simulink model "ES003A_PwrDiscnct"  (R2013b)
settings: Solver=ode45  StartTime=0.0  StopTime=5  RelTol=1e-3
values from neighbouring files (symbols this model uses):
  BattVltgSwdMax = DataDict.Calibration    [ES250A_BattVltg_DataDict.m]
  ELECGLBPRM_IVTRCNT_CNT_U08 = DataDict.ConfigParam    [ES999A_ElecGlbPrm_DataDict.m]
  PwrDiscnctNtc0x042FailStep = DataDict.Calibration    [ES003A_PwrDiscnct_DataDict.m]
  PwrDiscnctNtc0x042PassStep = DataDict.Calibration    [ES003A_PwrDiscnct_DataDict.m]
  PwrDiscnctNtc0x04AFailStep = DataDict.Calibration    [ES003A_PwrDiscnct_DataDict.m]
  PwrDiscnctNtc0x04APassStep = DataDict.Calibration    [ES003A_PwrDiscnct_DataDict.m]
  PwrDiscnctOpenThd = DataDict.Calibration    [ES003A_PwrDiscnct_DataDict.m]
libraries: simulink x1
settings Model: Creator=BZ9NJH  LastModifiedBy=BZ9NJH

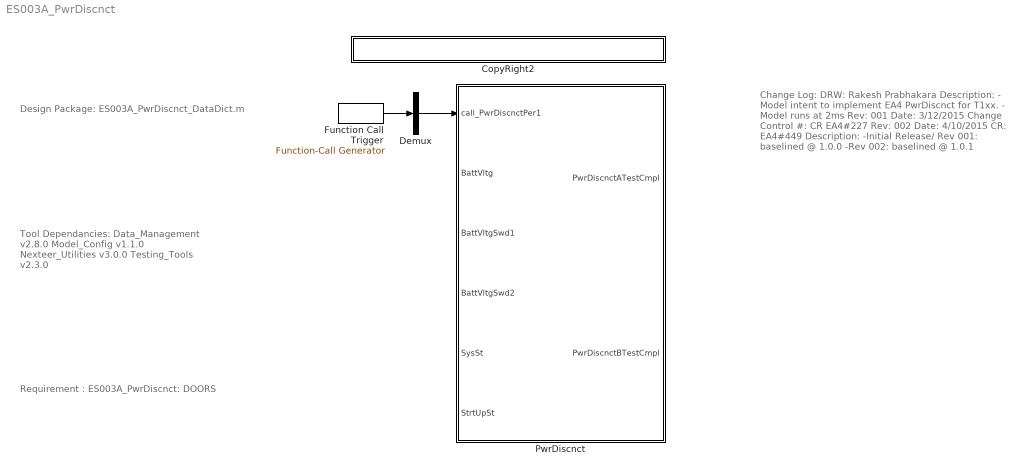
== system ES003A_PwrDiscnct ==
  note: Change Log:
      |
      | DRW: Rakesh Prabhakara
      | Description:
      | - Model intent to implement EA4 PwrDiscnct for T1xx.
      | - Model runs at 2ms
      |
      |
      | Rev: 001
      | Date: 3/12/2015
      | Change Control #: CR EA4#227
      |
      | Rev: 002
      | Date: 4/10/2015
      | CR: EA4#449
      |
      | Description:
      | -Initial Release/ Rev 001: baselined @ 1.0.0
      | -Rev 002: baselined @ 1.0.1
  note: Tool Dependancies:
      |
      | Data_Management v2.8.0
      | Model_Config v1.1.0
      | Nexteer_Utilities v3.0.0
      | Testing_Tools v2.3.0
  note: Design Package:
      |
      | ES003A_PwrDiscnct_DataDict.m
  note: Requirement :
      |
      | ES003A_PwrDiscnct: DOORS
  CopyRight2 : Subsystem  Description=|  mask(Copyright Information){none=on}
      | Copyright info block.                                               
      |                                                                     
      | Place copyright information at the top of every subsystem in design.
      mask prompts: none "No parameters"
      mask help: Place copyright information at the top of every subsystem in design.
      mask Display:
      | NxtrConf = 'Nexteer Confidential';
      | 
      | sys = bdroot; %handle for the current model ("system")
      | first = get_param(sys,'Created');
      | first = first(end-3:end);  %year is last four digits
      | 
      | last = get_param(sys,'LastModifiedDate');
      | if isempty(last)
      |     last = datestr(now,'yyyy');
      | else
      |     last = last(end-3:end);
      | end
      | 
      | if strcmp(first,last)
      |     fprintf('%s -- Copyright %s Nexteer',NxtrConf,first)
      | else
      |     fprintf('%s -- %s%s- %s Nexteer',NxtrConf,char(169),first,last)
      | end
  Demux : Demux  Outputs=1
  Function Call Trigger : simulink/Ports & Subsystems/Function-Call Generator  RequirementInfo={} %GIDa_15f970c6_0b7b_4174_a0b6_3f49a401e1d8  sample_time=0.002  numberOfIterations=1
  PwrDiscnct : Subsystem
  wires:
  Function Call Trigger/1 -> Demux/1
  Demux/1 -> PwrDiscnct/1(call_PwrDiscnctPer1)

== system ES003A_PwrDiscnct/CopyRight2 ==

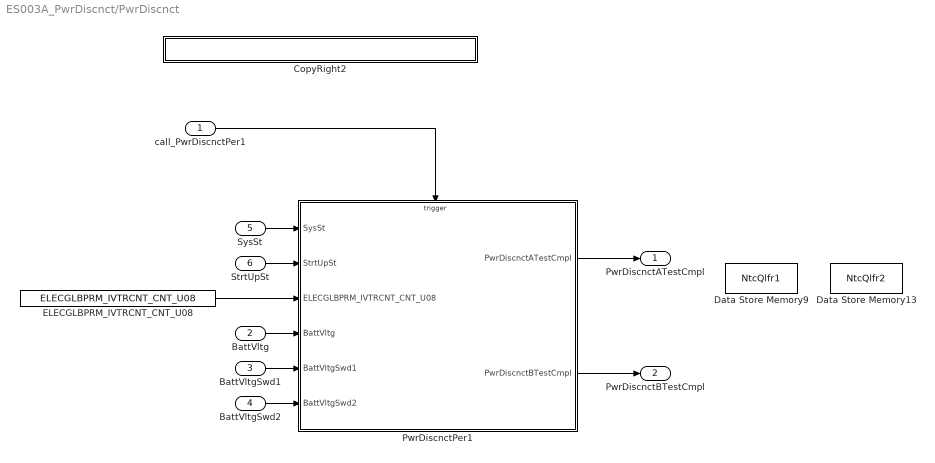
== system ES003A_PwrDiscnct/PwrDiscnct ==
  call_PwrDiscnctPer1 : Inport
  BattVltg : Inport  RequirementInfo={'linktype_rmi_doors' '0000c467 (/ESG Group/FDD Module Requirements/EA4 Specific/ES003A_PwrDiscnct)' '#ES003A_10' 'true' 'REQ: ES003A_10' '' } %GIDa_7969af00_7b99_4bd8_ab11_a14ecd32b67f  Port=2
  BattVltgSwd1 : Inport  RequirementInfo={'linktype_rmi_doors' '0000c467 (/ESG Group/FDD Module Requirements/EA4 Specific/ES003A_PwrDiscnct)' '#ES003A_11' 'true' 'REQ: ES003A_11' '' } %GIDa_b2ae44ec_3256_4720_9bec_d529845afe91  Port=3
  BattVltgSwd2 : Inport  RequirementInfo={'linktype_rmi_doors' '0000c467 (/ESG Group/FDD Module Requirements/EA4 Specific/ES003A_PwrDiscnct)' '#ES003A_12' 'true' 'REQ: ES003A_12' '' } %GIDa_6e68fbbb_22b3_47e1_b135_14c1a3669e24  Port=4
  SysSt : Inport  Port=5
  StrtUpSt : Inport  RequirementInfo={'linktype_rmi_doors' '0000c467 (/ESG Group/FDD Module Requirements/EA4 Specific/ES003A_PwrDiscnct)' '#ES003A_106' 'true' 'REQ: ES003A_106' '' } %GIDa_3a5ffb6b_2c5b_4987_b033_10885cd35b25  Port=6  OutDataTypeStr=double
  CopyRight2 : Subsystem  Description=|  mask(Copyright Information){none=on}
      | Copyright info block.                                               
      |                                                                     
      | Place copyright information at the top of every subsystem in design.
      mask prompts: none "No parameters"
      mask help: Place copyright information at the top of every subsystem in design.
      mask Display:
      | NxtrConf = 'Nexteer Confidential';
      | 
      | sys = bdroot; %handle for the current model ("system")
      | first = get_param(sys,'Created');
      | first = first(end-3:end);  %year is last four digits
      | 
      | last = get_param(sys,'LastModifiedDate');
      | if isempty(last)
      |     last = datestr(now,'yyyy');
      | else
      |     last = last(end-3:end);
      | end
      | 
      | if strcmp(first,last)
      |     fprintf('%s -- Copyright %s Nexteer',NxtrConf,first)
      | else
      |     fprintf('%s -- %s%s- %s Nexteer',NxtrConf,char(169),first,last)
      | end
  Data Store Memory13 : DataStoreMemory  DataStoreName=NtcQlfr2  ReadBeforeWriteMsg=warning  WriteAfterWriteMsg=warning  WriteAfterReadMsg=warning
  Data Store Memory9 : DataStoreMemory  DataStoreName=NtcQlfr1  ReadBeforeWriteMsg=warning  WriteAfterWriteMsg=warning  WriteAfterReadMsg=warning
  ELECGLBPRM_IVTRCNT_CNT_U08 : Constant  RequirementInfo={'linktype_rmi_doors' '0000c467 (/ESG Group/FDD Module Requirements/EA4 Specific/ES003A_PwrDiscnct)' '#ES003A_13' 'true' 'REQ: ES003A_13' '' } %GIDa_8c2aeced_6f98_4fdd_a2dd_374f750473e0  Value=ELECGLBPRM_IVTRCNT_CNT_U08  OutDataTypeStr=single
  PwrDiscnctPer1 : Subsystem  RequirementInfo={'linktype_rmi_doors' '0000c467 (/ESG Group/FDD Module Requirements/EA4 Specific/ES003A_PwrDiscnct)' '#ES003A_98' 'true' 'REQ: ES003A_98' '' } %GIDa_d6496f46_22fb_4d18_9ef4_8fee2b8599d6  TreatAsAtomicUnit=on
  PwrDiscnctATestCmpl : Outport  RequirementInfo={'linktype_rmi_doors' '0000c467 (/ESG Group/FDD Module Requirements/EA4 Specific/ES003A_PwrDiscnct)' '#ES003A_15' 'true' 'REQ: ES003A_15' '' } %GIDa_a54f22bb_d830_4888_91ed_92219a6abd25
  PwrDiscnctBTestCmpl : Outport  RequirementInfo={'linktype_rmi_doors' '0000c467 (/ESG Group/FDD Module Requirements/EA4 Specific/ES003A_PwrDiscnct)' '#ES003A_14' 'true' 'REQ: ES003A_14' '' } %GIDa_e99709b4_314c_405c_b628_2ebeb252bf18  Port=2
  wires:
  call_PwrDiscnctPer1/1 -> PwrDiscnctPer1/Trigger
  PwrDiscnctPer1/1(PwrDiscnctATestCmpl) -> PwrDiscnctATestCmpl/1
  PwrDiscnctPer1/2(PwrDiscnctBTestCmpl) -> PwrDiscnctBTestCmpl/1
  StrtUpSt/1 -> PwrDiscnctPer1/2(StrtUpSt)
  SysSt/1 -> PwrDiscnctPer1/1(SysSt)
  ELECGLBPRM_IVTRCNT_CNT_U08/1 -> PwrDiscnctPer1/3(ELECGLBPRM_IVTRCNT_CNT_U08)
  BattVltg/1 -> PwrDiscnctPer1/4(BattVltg)
  BattVltgSwd2/1 -> PwrDiscnctPer1/6(BattVltgSwd2)
  BattVltgSwd1/1 -> PwrDiscnctPer1/5(BattVltgSwd1)

== system ES003A_PwrDiscnct/PwrDiscnct/CopyRight2 ==

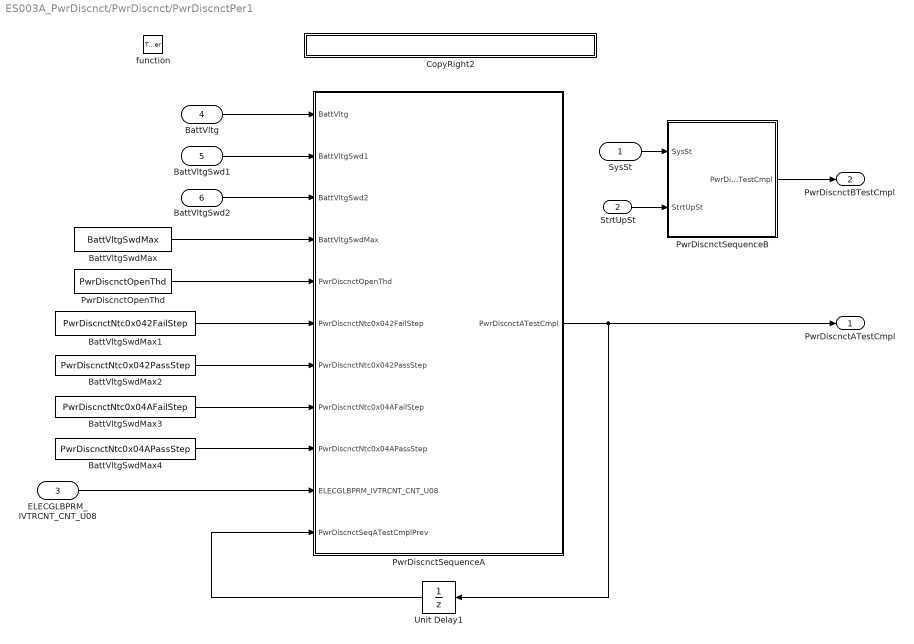
== system ES003A_PwrDiscnct/PwrDiscnct/PwrDiscnctPer1 ==
  SysSt : Inport
  StrtUpSt : Inport  Port=2  OutDataTypeStr=double
  ELECGLBPRM_IVTRCNT_CNT_U08 : Inport  Port=3
  BattVltg : Inport  Port=4
  BattVltgSwd1 : Inport  Port=5
  BattVltgSwd2 : Inport  Port=6
  function : TriggerPort  TriggerType=function-call
  BattVltgSwdMax : Constant  RequirementInfo={'linktype_rmi_doors' '0000c467 (/ESG Group/FDD Module Requirements/EA4 Specific/ES003A_PwrDiscnct)' '#ES003A_18' 'true' 'REQ: ES003A_18' '' } %GIDa_75c0cbae_266b_43df_b9ef_273f9bdf4671  Value=BattVltgSwdMax
  BattVltgSwdMax1 : Constant  Value=PwrDiscnctNtc0x042FailStep
  BattVltgSwdMax2 : Constant  Value=PwrDiscnctNtc0x042PassStep
  BattVltgSwdMax3 : Constant  Value=PwrDiscnctNtc0x04AFailStep
  BattVltgSwdMax4 : Constant  Value=PwrDiscnctNtc0x04APassStep
  CopyRight2 : Subsystem  Description=|  mask(Copyright Information){none=on}
      | Copyright info block.                                               
      |                                                                     
      | Place copyright information at the top of every subsystem in design.
      mask prompts: none "No parameters"
      mask help: Place copyright information at the top of every subsystem in design.
      mask Display:
      | NxtrConf = 'Nexteer Confidential';
      | 
      | sys = bdroot; %handle for the current model ("system")
      | first = get_param(sys,'Created');
      | first = first(end-3:end);  %year is last four digits
      | 
      | last = get_param(sys,'LastModifiedDate');
      | if isempty(last)
      |     last = datestr(now,'yyyy');
      | else
      |     last = last(end-3:end);
      | end
      | 
      | if strcmp(first,last)
      |     fprintf('%s -- Copyright %s Nexteer',NxtrConf,first)
      | else
      |     fprintf('%s -- %s%s- %s Nexteer',NxtrConf,char(169),first,last)
      | end
  PwrDiscnctOpenThd : Constant  RequirementInfo={'linktype_rmi_doors' '0000c467 (/ESG Group/FDD Module Requirements/EA4 Specific/ES003A_PwrDiscnct)' '#ES003A_22' 'true' 'REQ: ES003A_22' '' } %GIDa_a84f9b62_e1cf_4caf_a19c_8d6c01e9295c  Value=PwrDiscnctOpenThd
  PwrDiscnctSequenceA : Stateflow chart  RequirementInfo={'linktype_rmi_doors' '0000c467 (/ESG Group/FDD Module Requirements/EA4 Specific/ES003A_PwrDiscnct)' '#ES003A_47' 'true' 'REQ: ES003A_47' '' } %GIDa_3ade2cbb_cb37_4d62_9bbf_15e89d094b58  TreatAsAtomicUnit=on
  PwrDiscnctSequenceB : Subsystem  RequirementInfo={'linktype_rmi_doors' '0000c467 (/ESG Group/FDD Module Requirements/EA4 Specific/ES003A_PwrDiscnct)' '#ES003A_82' 'true' 'REQ: ES003A_82' '' ; 'linktype_rmi_doors' '0000c467 (/ESG Group/FDD Module Requirements/EA4 Specific/ES003A_PwrDiscnct)' '#ES003A_88' 'true' 'REQ: ES003A_88' '' } %GIDa_af92003a_7581_41aa_9d02_d4566cd9fce6
  Unit Delay1 : UnitDelay  SampleTime=-1  StateName=PwrDiscnctSeqATestCmplPrev  StateMustResolveToSignalObject=on
      settings: AttributesFormatString=|
      | State Name:
      | %<StateName>
  PwrDiscnctATestCmpl : Outport
  PwrDiscnctBTestCmpl : Outport  Port=2
  wires:
  SysSt/1 -> PwrDiscnctSequenceB/1(SysSt)
  BattVltg/1 -> PwrDiscnctSequenceA/1(BattVltg)
  BattVltgSwd1/1 -> PwrDiscnctSequenceA/2(BattVltgSwd1)
  BattVltgSwd2/1 -> PwrDiscnctSequenceA/3(BattVltgSwd2)
  ELECGLBPRM_IVTRCNT_CNT_U08/1 -> PwrDiscnctSequenceA/10(ELECGLBPRM_IVTRCNT_CNT_U08)
  PwrDiscnctOpenThd/1 -> PwrDiscnctSequenceA/5(PwrDiscnctOpenThd)
  BattVltgSwdMax/1 -> PwrDiscnctSequenceA/4(BattVltgSwdMax)
  BattVltgSwdMax1/1 -> PwrDiscnctSequenceA/6(PwrDiscnctNtc0x042FailStep)
  BattVltgSwdMax2/1 -> PwrDiscnctSequenceA/7(PwrDiscnctNtc0x042PassStep)
  BattVltgSwdMax3/1 -> PwrDiscnctSequenceA/8(PwrDiscnctNtc0x04AFailStep)
  BattVltgSwdMax4/1 -> PwrDiscnctSequenceA/9(PwrDiscnctNtc0x04APassStep)
  PwrDiscnctSequenceA/1(PwrDiscnctATestCmpl) -> Unit Delay1/1, PwrDiscnctATestCmpl/1
  Unit Delay1/1 -> PwrDiscnctSequenceA/11(PwrDiscnctSeqATestCmplPrev)
  PwrDiscnctSequenceB/1(PwrDiscnctBTestCmpl) -> PwrDiscnctBTestCmpl/1
  StrtUpSt/1 -> PwrDiscnctSequenceB/2(StrtUpSt)

== system ES003A_PwrDiscnct/PwrDiscnct/PwrDiscnctPer1/CopyRight2 ==

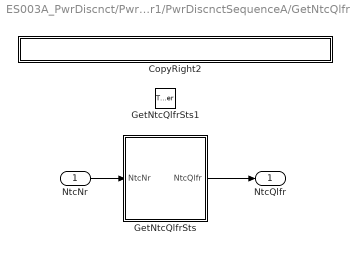
== system ES003A_PwrDiscnct/PwrDiscnct/PwrDiscnctPer1/PwrDiscnctSequenceA/GetNtcQlfrSts ==
  NtcNr : Inport  OutDataTypeStr=int16  PortDimensions=1
  GetNtcQlfrSts1 : TriggerPort  TriggerType=function-call
      settings: CopyFcn=Stateflow.SLINSF.SimulinkMan.removeBlockPreDeleteFcn  PreDeleteFcn=Stateflow.SLINSF.SimulinkMan.unsafePredeleteFcn
  CopyRight2 : Subsystem  Description=|  mask(Copyright Information){none=on}
      | Copyright info block.                                               
      |                                                                     
      | Place copyright information at the top of every subsystem in design.
      mask prompts: none "No parameters"
      mask help: Place copyright information at the top of every subsystem in design.
      mask Display:
      | NxtrConf = 'Nexteer Confidential';
      | 
      | sys = bdroot; %handle for the current model ("system")
      | first = get_param(sys,'Created');
      | first = first(end-3:end);  %year is last four digits
      | 
      | last = get_param(sys,'LastModifiedDate');
      | if isempty(last)
      |     last = datestr(now,'yyyy');
      | else
      |     last = last(end-3:end);
      | end
      | 
      | if strcmp(first,last)
      |     fprintf('%s -- Copyright %s Nexteer',NxtrConf,first)
      | else
      |     fprintf('%s -- %s%s- %s Nexteer',NxtrConf,char(169),first,last)
      | end
  GetNtcQlfrSts : Subsystem  RequirementInfo={} %GIDa_55b4ee3c_edbf_4f51_ae1c_660e8f62e0b1  TreatAsAtomicUnit=on
      settings: RTWSystemCode=Inline
  NtcQlfr : Outport
  wires:
  NtcNr/1 -> GetNtcQlfrSts/1(NtcNr)
  GetNtcQlfrSts/1(NtcQlfr) -> NtcQlfr/1

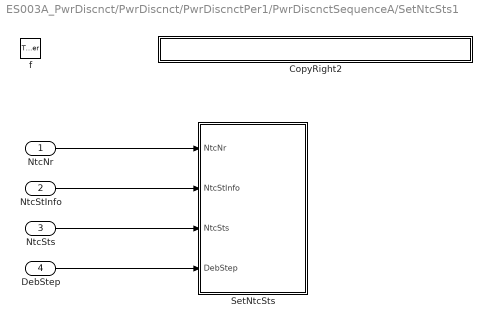
== system ES003A_PwrDiscnct/PwrDiscnct/PwrDiscnctPer1/PwrDiscnctSequenceA/SetNtcSts1 ==
  NtcNr : Inport  PortDimensions=1
  NtcStInfo : Inport  Port=2  PortDimensions=1
  NtcSts : Inport  Port=3  PortDimensions=1
  DebStep : Inport  Port=4  PortDimensions=1
  f : TriggerPort  TriggerType=function-call
      settings: CopyFcn=Stateflow.SLINSF.SimulinkMan.removeBlockPreDeleteFcn  PreDeleteFcn=Stateflow.SLINSF.SimulinkMan.unsafePredeleteFcn
  CopyRight2 : Subsystem  Description=|  mask(Copyright Information){none=on}
      | Copyright info block.                                               
      |                                                                     
      | Place copyright information at the top of every subsystem in design.
      mask prompts: none "No parameters"
      mask help: Place copyright information at the top of every subsystem in design.
      mask Display:
      | NxtrConf = 'Nexteer Confidential';
      | 
      | sys = bdroot; %handle for the current model ("system")
      | first = get_param(sys,'Created');
      | first = first(end-3:end);  %year is last four digits
      | 
      | last = get_param(sys,'LastModifiedDate');
      | if isempty(last)
      |     last = datestr(now,'yyyy');
      | else
      |     last = last(end-3:end);
      | end
      | 
      | if strcmp(first,last)
      |     fprintf('%s -- Copyright %s Nexteer',NxtrConf,first)
      | else
      |     fprintf('%s -- %s%s- %s Nexteer',NxtrConf,char(169),first,last)
      | end
  SetNtcSts : Subsystem  RequirementInfo={} %GIDa_82714b20_8369_498a_a3bf_ae484680a262  VariantControl=NTC_sim
  wires:
  NtcStInfo/1 -> SetNtcSts/2(NtcStInfo)
  NtcNr/1 -> SetNtcSts/1(NtcNr)
  NtcSts/1 -> SetNtcSts/3(NtcSts)
  DebStep/1 -> SetNtcSts/4(DebStep)

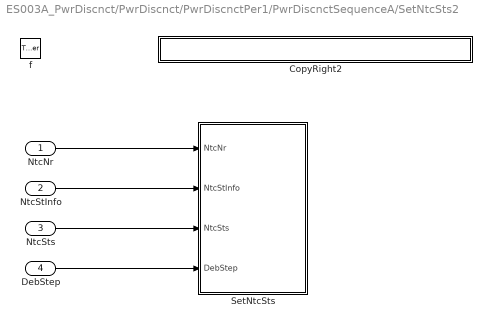
== system ES003A_PwrDiscnct/PwrDiscnct/PwrDiscnctPer1/PwrDiscnctSequenceA/SetNtcSts2 ==
  NtcNr : Inport  PortDimensions=1
  NtcStInfo : Inport  Port=2  PortDimensions=1
  NtcSts : Inport  Port=3  PortDimensions=1
  DebStep : Inport  Port=4  PortDimensions=1
  f : TriggerPort  TriggerType=function-call
      settings: CopyFcn=Stateflow.SLINSF.SimulinkMan.removeBlockPreDeleteFcn  PreDeleteFcn=Stateflow.SLINSF.SimulinkMan.unsafePredeleteFcn
  CopyRight2 : Subsystem  Description=|  mask(Copyright Information){none=on}
      | Copyright info block.                                               
      |                                                                     
      | Place copyright information at the top of every subsystem in design.
      mask prompts: none "No parameters"
      mask help: Place copyright information at the top of every subsystem in design.
      mask Display:
      | NxtrConf = 'Nexteer Confidential';
      | 
      | sys = bdroot; %handle for the current model ("system")
      | first = get_param(sys,'Created');
      | first = first(end-3:end);  %year is last four digits
      | 
      | last = get_param(sys,'LastModifiedDate');
      | if isempty(last)
      |     last = datestr(now,'yyyy');
      | else
      |     last = last(end-3:end);
      | end
      | 
      | if strcmp(first,last)
      |     fprintf('%s -- Copyright %s Nexteer',NxtrConf,first)
      | else
      |     fprintf('%s -- %s%s- %s Nexteer',NxtrConf,char(169),first,last)
      | end
  SetNtcSts : Subsystem  RequirementInfo={} %GIDa_0f1cc213_d07f_475f_8cac_6a7fd5400116  VariantControl=NTC_sim
  wires:
  NtcStInfo/1 -> SetNtcSts/2(NtcStInfo)
  NtcNr/1 -> SetNtcSts/1(NtcNr)
  NtcSts/1 -> SetNtcSts/3(NtcSts)
  DebStep/1 -> SetNtcSts/4(DebStep)

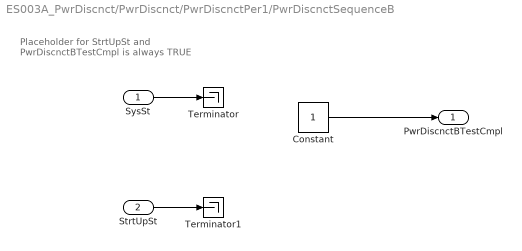
== system ES003A_PwrDiscnct/PwrDiscnct/PwrDiscnctPer1/PwrDiscnctSequenceB ==
  note: Placeholder for StrtUpSt
      | and  PwrDiscnctBTestCmpl is always TRUE
  SysSt : Inport
  StrtUpSt : Inport  Port=2
  Constant : Constant
  Terminator : Terminator
  Terminator1 : Terminator
  PwrDiscnctBTestCmpl : Outport
  wires:
  Constant/1 -> PwrDiscnctBTestCmpl/1
  SysSt/1 -> Terminator/1
  StrtUpSt/1 -> Terminator1/1

== system ES003A_PwrDiscnct/PwrDiscnct/PwrDiscnctPer1/PwrDiscnctSequenceA/GetNtcQlfrSts/CopyRight2 ==

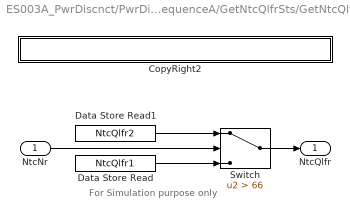
== system ES003A_PwrDiscnct/PwrDiscnct/PwrDiscnctPer1/PwrDiscnctSequenceA/GetNtcQlfrSts/GetNtcQlfrSts ==
  note: For Simulation purpose only
  NtcNr : Inport
  CopyRight2 : Subsystem  Description=|  mask(Copyright Information){none=on}
      | Copyright info block.                                               
      |                                                                     
      | Place copyright information at the top of every subsystem in design.
      mask prompts: none "No parameters"
      mask help: Place copyright information at the top of every subsystem in design.
      mask Display:
      | NxtrConf = 'Nexteer Confidential';
      | 
      | sys = bdroot; %handle for the current model ("system")
      | first = get_param(sys,'Created');
      | first = first(end-3:end);  %year is last four digits
      | 
      | last = get_param(sys,'LastModifiedDate');
      | if isempty(last)
      |     last = datestr(now,'yyyy');
      | else
      |     last = last(end-3:end);
      | end
      | 
      | if strcmp(first,last)
      |     fprintf('%s -- Copyright %s Nexteer',NxtrConf,first)
      | else
      |     fprintf('%s -- %s%s- %s Nexteer',NxtrConf,char(169),first,last)
      | end
  Data Store Read : DataStoreRead  DataStoreName=NtcQlfr1
  Data Store Read1 : DataStoreRead  DataStoreName=NtcQlfr2
  Switch : Switch  Criteria=u2 > Threshold  Threshold=66
  NtcQlfr : Outport
  wires:
  Switch/1 -> NtcQlfr/1
  NtcNr/1 -> Switch/2
  Data Store Read1/1 -> Switch/1
  Data Store Read/1 -> Switch/3

== system ES003A_PwrDiscnct/PwrDiscnct/PwrDiscnctPer1/PwrDiscnctSequenceA/SetNtcSts1/CopyRight2 ==

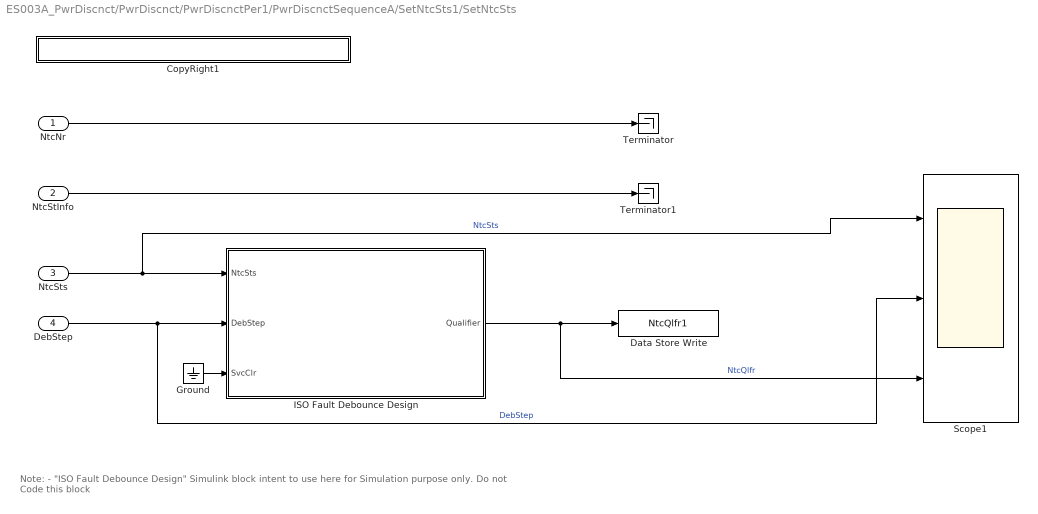
== system ES003A_PwrDiscnct/PwrDiscnct/PwrDiscnctPer1/PwrDiscnctSequenceA/SetNtcSts1/SetNtcSts ==
  note: Note:
      |
      | - "ISO Fault Debounce Design" Simulink block intent to use here for Simulation purpose only. Do not Code this block
  NtcNr : Inport
  NtcStInfo : Inport  Port=2
  NtcSts : Inport  Port=3
  DebStep : Inport  Port=4
  CopyRight1 : Subsystem  Description=|  mask(Copyright Information){none=on}
      | Copyright info block.                                               
      |                                                                     
      | Place copyright information at the top of every subsystem in design.
      mask prompts: none "No parameters"
      mask help: Place copyright information at the top of every subsystem in design.
      mask Display:
      | NxtrConf = 'Nexteer Confidential';
      | 
      | sys = bdroot; %handle for the current model ("system")
      | first = get_param(sys,'Created');
      | first = first(end-3:end);  %year is last four digits
      | 
      | last = get_param(sys,'LastModifiedDate');
      | if isempty(last)
      |     last = datestr(now,'yyyy');
      | else
      |     last = last(end-3:end);
      | end
      | 
      | if strcmp(first,last)
      |     fprintf('%s -- Copyright %s Nexteer',NxtrConf,first)
      | else
      |     fprintf('%s -- %s%s- %s Nexteer',NxtrConf,char(169),first,last)
      | end
  Data Store Write : DataStoreWrite  DataStoreName=NtcQlfr1
  Ground : Ground
  ISO Fault Debounce Design : Stateflow chart  TreatAsAtomicUnit=on
      settings: AttributesFormatString=|
      | Simulation Purpose Only.
      | Do Not Code this block
      | Diagnostic Manager Owns this requirement
  Scope1 : Scope  NumInputPorts=3
      settings: YMin=1.9~3891.2~-1  YMax=2.1~4300.8~1
  Terminator : Terminator
  Terminator1 : Terminator
  wires:
  NtcStInfo/1 -> Terminator1/1
  NtcNr/1 -> Terminator/1
  NtcSts/1 -> ISO Fault Debounce Design/1(NtcSts), Scope1/1  "NtcSts"
  DebStep/1 -> ISO Fault Debounce Design/2(DebStep), Scope1/2  "DebStep"
  ISO Fault Debounce Design/1(Qualifier) -> Scope1/3, Data Store Write/1  "NtcQlfr"
  Ground/1 -> ISO Fault Debounce Design/3(SvcClr)

== system ES003A_PwrDiscnct/PwrDiscnct/PwrDiscnctPer1/PwrDiscnctSequenceA/SetNtcSts2/CopyRight2 ==

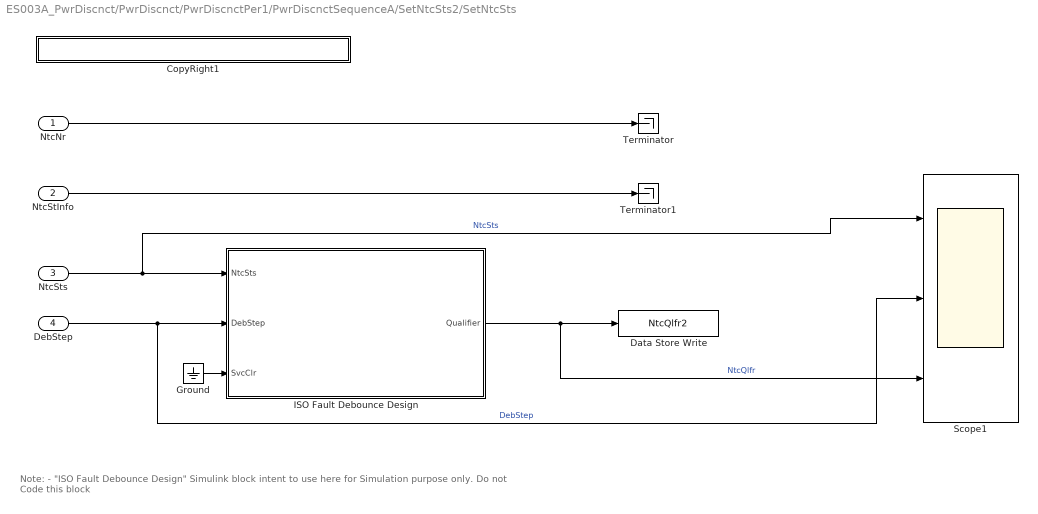
== system ES003A_PwrDiscnct/PwrDiscnct/PwrDiscnctPer1/PwrDiscnctSequenceA/SetNtcSts2/SetNtcSts ==
  note: Note:
      |
      | - "ISO Fault Debounce Design" Simulink block intent to use here for Simulation purpose only. Do not Code this block
  NtcNr : Inport
  NtcStInfo : Inport  Port=2
  NtcSts : Inport  Port=3
  DebStep : Inport  Port=4
  CopyRight1 : Subsystem  Description=|  mask(Copyright Information){none=on}
      | Copyright info block.                                               
      |                                                                     
      | Place copyright information at the top of every subsystem in design.
      mask prompts: none "No parameters"
      mask help: Place copyright information at the top of every subsystem in design.
      mask Display:
      | NxtrConf = 'Nexteer Confidential';
      | 
      | sys = bdroot; %handle for the current model ("system")
      | first = get_param(sys,'Created');
      | first = first(end-3:end);  %year is last four digits
      | 
      | last = get_param(sys,'LastModifiedDate');
      | if isempty(last)
      |     last = datestr(now,'yyyy');
      | else
      |     last = last(end-3:end);
      | end
      | 
      | if strcmp(first,last)
      |     fprintf('%s -- Copyright %s Nexteer',NxtrConf,first)
      | else
      |     fprintf('%s -- %s%s- %s Nexteer',NxtrConf,char(169),first,last)
      | end
  Data Store Write : DataStoreWrite  DataStoreName=NtcQlfr2
  Ground : Ground
  ISO Fault Debounce Design : Stateflow chart  TreatAsAtomicUnit=on
      settings: AttributesFormatString=|
      | Simulation Purpose Only.
      | Do Not Code this block
      | Diagnostic Manager Owns this requirement
  Scope1 : Scope  NumInputPorts=3
      settings: YMin=1.9~486.4~0  YMax=2.1~537.6~1
  Terminator : Terminator
  Terminator1 : Terminator
  wires:
  NtcStInfo/1 -> Terminator1/1
  NtcNr/1 -> Terminator/1
  NtcSts/1 -> ISO Fault Debounce Design/1(NtcSts), Scope1/1  "NtcSts"
  DebStep/1 -> ISO Fault Debounce Design/2(DebStep), Scope1/2  "DebStep"
  ISO Fault Debounce Design/1(Qualifier) -> Scope1/3, Data Store Write/1  "NtcQlfr"
  Ground/1 -> ISO Fault Debounce Design/3(SvcClr)

== system ES003A_PwrDiscnct/PwrDiscnct/PwrDiscnctPer1/PwrDiscnctSequenceA/GetNtcQlfrSts/GetNtcQlfrSts/CopyRight2 ==

== system ES003A_PwrDiscnct/PwrDiscnct/PwrDiscnctPer1/PwrDiscnctSequenceA/SetNtcSts1/SetNtcSts/CopyRight1 ==

== system ES003A_PwrDiscnct/PwrDiscnct/PwrDiscnctPer1/PwrDiscnctSequenceA/SetNtcSts2/SetNtcSts/CopyRight1 ==

== stateflow chart ES003A_PwrDiscnct/PwrDiscnct/PwrDiscnctPer1/PwrDiscnctSequenceA ==
  state SetNtcSts1(NtcNr, NtcStInfo, NtcSts, DebStep) [function]
  state NtcQlfr = GetNtcQlfrSts(NtcNr) [function]
  state SetNtcSts2(NtcNr, NtcStInfo, NtcSts, DebStep) [function]
  (default) -> (junction 29)
  (junction 29) -> (junction 112) [order 1] : [PwrDiscnctSeqATestCmplPrev == 0]
      | {PwrDiscnctDeltaVltg1 =abs(min(BattVltgSwdMax, BattVltg) - BattVltgSwd1);}
  (junction 112) -> (junction 34) [order 1] : [PwrDiscnctDeltaVltg1 >= PwrDiscnctOpenThd]
      | {SetNtcSts1(NTCNR_0X042, 0, 2, PwrDiscnctNtc0x042PassStep);}
  (junction 112) -> (junction 34) [order 2] : {SetNtcSts1(NTCNR_0X042,0,3,PwrDiscnctNtc0x042FailStep);}
  (junction 29) -> (junction 113) [order 2] : {PwrDiscnctATestCmpl = 1;}
  (junction 80) -> (junction 113) [order 2] : {PwrDiscnctATestCmpl = 0;}
  (junction 80) -> (junction 113) [order 1] : [PwrDiscnct1Qlfr  > 0]
      | {PwrDiscnctATestCmpl = 1;}
  (junction 34) -> (junction 80) [order 2] : {PwrDiscnct1Qlfr = GetNtcQlfrSts(NTCNR_0X042)}
  (junction 81) -> (junction 113) [order 1] : [PwrDiscnct1Qlfr  > 0 &&  PwrDiscnct2Qlfr > 0]
      | {PwrDiscnctATestCmpl = 1;}
  (junction 34) -> (junction 111) [order 1] : [ELECGLBPRM_IVTRCNT_CNT_U08 == 2]
      | {PwrDiscnctDeltaVltg2= abs(min(BattVltgSwdMax, BattVltg) - BattVltgSwd2);}
  (junction 81) -> (junction 113) [order 2] : {PwrDiscnctATestCmpl = 0;}
  (junction 111) -> (junction 8) [order 1] : [PwrDiscnctDeltaVltg2 >= PwrDiscnctOpenThd]
      | {SetNtcSts2(NTCNR_0X04A,0,2,PwrDiscnctNtc0x04APassStep);}
  (junction 111) -> (junction 8) [order 2] : {SetNtcSts2(NTCNR_0X04A,0,3,PwrDiscnctNtc0x04AFailStep);}
  (junction 8) -> (junction 81) : {
      | PwrDiscnct1Qlfr = GetNtcQlfrSts(NTCNR_0X042);
      | PwrDiscnct2Qlfr = GetNtcQlfrSts(NTCNR_0X04A);
      | }
  data: NtcNr function_input size=1; NtcStInfo function_input size=1; NtcSts function_input size=1; DebStep function_input size=1; NtcNr function_input int16 size=1; NtcQlfr function_output; NtcNr function_input size=1; NtcStInfo function_input size=1; NtcSts function_input size=1; DebStep function_input size=1; BattVltg input; BattVltgSwd1 input; BattVltgSwd2 input; BattVltgSwdMax input; NtcQlfr0x042 local uint8; NtcQlfr0x04A local uint8; PwrDiscnctOpenThd input; PwrDiscnctATestCmpl output boolean; PwrDiscnct1Qlfr local uint8; PwrDiscnct2Qlfr local uint8; PwrDiscnctNtc0x042FailStep input; PwrDiscnctNtc0x042PassStep input; PwrDiscnctNtc0x04AFailStep input; PwrDiscnctNtc0x04APassStep input; PwrDiscnctDeltaVltg1 local int16; PwrDiscnctDeltaVltg2 local int16; ELECGLBPRM_IVTRCNT_CNT_U08 input; PwrDiscnctSeqATestCmplPrev input; NTCNR_0X042 local uint16 =66; NTCNR_0X04A local uint16 =74

== stateflow chart ES003A_PwrDiscnct/PwrDiscnct/PwrDiscnctPer1/PwrDiscnctSequenceA/SetNtcSts1/SetNtcSts/ISO Fault Debounce Design ==
  note: NTCSTS_PASSD           (0)
      | NTCSTS_FAILD             (1)
      | NTCSTS_PREPASSD   (2)
      | NTCSTS_PREFAILD     (3)
      |
      | SIGQLFR_NORES        (0)
      | SIGQLFR_PASSD         (1)
      | SIGQLFR_FAILD           (2)
  note: Pass Loop
  note: Fail Loop
  note: 
  (default) -> (junction 89)
  (junction 89) -> (junction 95) [order 1] : [NtcSts ==3]
  (junction 89) -> (junction 93) [order 2]
  (junction 89) -> (junction 141) [order 3] : [NtcSts ==1]
      | { ErrAcc = 32767;
      | Qualifier =2;
      |  }
  (junction 89) -> (junction 141) [order 4] : [NtcSts ==0]
      | { ErrAcc = -32768;
      | Qualifier=1;
      | }
  (junction 95) -> (junction 103) [order 2]
  (junction 95) -> (junction 111) [order 1] : [ErrAcc <=0]
      | {ErrAcc = DebStep;}
  (junction 93) -> (junction 123) [order 2] : {
      | ErrAcc = ErrAcc - DebStep;
      | }
  (junction 93) -> (junction 123) [order 1] : [(ErrAcc - DebStep) <= -32768]
      | { ErrAcc = -32768;
      | Qualifier=1;
      | }
  (junction 103) -> (junction 111) [order 1] : [(ErrAcc + DebStep) <32767]
      | {ErrAcc = ErrAcc + DebStep;}
  (junction 103) -> (junction 111) [order 2] : {ErrAcc = 32767;
      | Qualifier =2;}
  (junction 123) -> (junction 141)
  (junction 111) -> (junction 141)
  (junction 141) -> (junction 159) [order 2] : [SvcClr ==1]
      | {ErrAcc = 0;
      | Qualifier =0;
      | }
  (junction 141) -> (junction 159) [order 1]
  data: NtcSts input uint8; Qualifier output uint8; DebStep input int32; ErrAcc local int16; SvcClr input

== stateflow chart ES003A_PwrDiscnct/PwrDiscnct/PwrDiscnctPer1/PwrDiscnctSequenceA/SetNtcSts2/SetNtcSts/ISO Fault Debounce Design ==
  note: NTCSTS_PASSD           (0)
      | NTCSTS_FAILD             (1)
      | NTCSTS_PREPASSD   (2)
      | NTCSTS_PREFAILD     (3)
      |
      | SIGQLFR_NORES        (0)
      | SIGQLFR_PASSD         (1)
      | SIGQLFR_FAILD           (2)
  note: Pass Loop
  note: Fail Loop
  note: 
  (default) -> (junction 89)
  (junction 89) -> (junction 95) [order 1] : [NtcSts ==3]
  (junction 89) -> (junction 93) [order 2]
  (junction 89) -> (junction 141) [order 3] : [NtcSts ==1]
      | { ErrAcc = 32767;
      | Qualifier =2;
      |  }
  (junction 89) -> (junction 141) [order 4] : [NtcSts ==0]
      | { ErrAcc = -32768;
      | Qualifier=1;
      | }
  (junction 95) -> (junction 103) [order 2]
  (junction 95) -> (junction 111) [order 1] : [ErrAcc <=0]
      | {ErrAcc = DebStep;}
  (junction 93) -> (junction 123) [order 2] : {
      | ErrAcc = ErrAcc - DebStep;
      | }
  (junction 93) -> (junction 123) [order 1] : [(ErrAcc - DebStep) <= -32768]
      | { ErrAcc = -32768;
      | Qualifier=1;
      | }
  (junction 103) -> (junction 111) [order 1] : [(ErrAcc + DebStep) <32767]
      | {ErrAcc = ErrAcc + DebStep;}
  (junction 103) -> (junction 111) [order 2] : {ErrAcc = 32767;
      | Qualifier =2;}
  (junction 123) -> (junction 141)
  (junction 111) -> (junction 141)
  (junction 141) -> (junction 159) [order 2] : [SvcClr ==1]
      | {ErrAcc = 0;
      | Qualifier =0;
      | }
  (junction 141) -> (junction 159) [order 1]
  data: NtcSts input uint8; Qualifier output uint8; DebStep input int32; ErrAcc local int16; SvcClr input
